simulink model "leftcameraagent"  (Simulink 6.2)
settings: Solver=ode45  StartTime=0.0  StopTime=10.0  RelTol=1e-3
settings Model: LastModifiedBy=suarezjl
settings DataIOCC: SignalLoggingName=sigsOut
settings HardwareCC: TargetUnknown=on

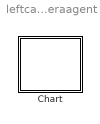
== system leftcameraagent ==
  Chart : Stateflow chart

== stateflow chart Chart ==
  state Initial
    \\Sally\LeftReachDemo\HeadModule\LeftCameraAgent\FrameGrabber.Initialize()
    \\Sally\LeftReachDemo\HeadModule\LeftCameraAgent\FrameGrabber.ObtainImage()
    \\Sally\LeftReachDemo\HeadModule\LeftCameraAgent\FrameGrabber.ObtainImage()
    \\Sally\LeftReachDemo\HeadModule\LeftCameraAgent\ColorSegmenter.Initial()
    \\Sally\LeftReachDemo\HeadModule\LeftCameraAgent\ColorSegmenter.LoadColorModel()
  state Segmentation
    \\Sally\LeftReachDemo\HeadModule\LeftCameraAgent\FrameGrabber.ObtainImage()
    \\Sally\LeftReachDemo\HeadModule\LeftCameraAgent\ColorSegmenter.DoSegment()
  (default) -> Initial : Start
  Initial -> Segmentation : Always
  Segmentation -> Segmentation : Always
